simulink model "FlightCore_ROS2_loop"  (R2025b)
settings: Solver=FixedStepDiscrete  StartTime=0.0  StopTime=120  FixedStep=0.001  RelTol=1e-3
undefined symbols (not defined in the file): accel_bias_mps2, accel_body_mps2, angular_rate_body_radps, attitude_quat_wxyz, gyro_bias_radps, motor_cmd, position_ned_m, sequence, source_id, status, timestamp_sec, valid, velocity_ned_mps, wind_ned_mps
libraries: ros2lib x6
settings Model: DataDictionary=GlobalTypes.sldd  Creator=89447  LastModifiedBy=89447

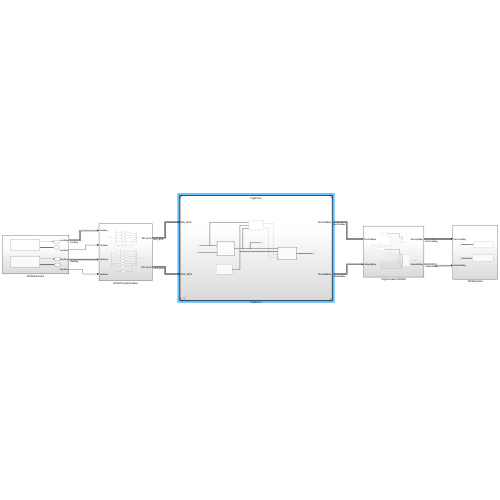
[thumbnail: Simulink's stored preview of the top-level diagram]
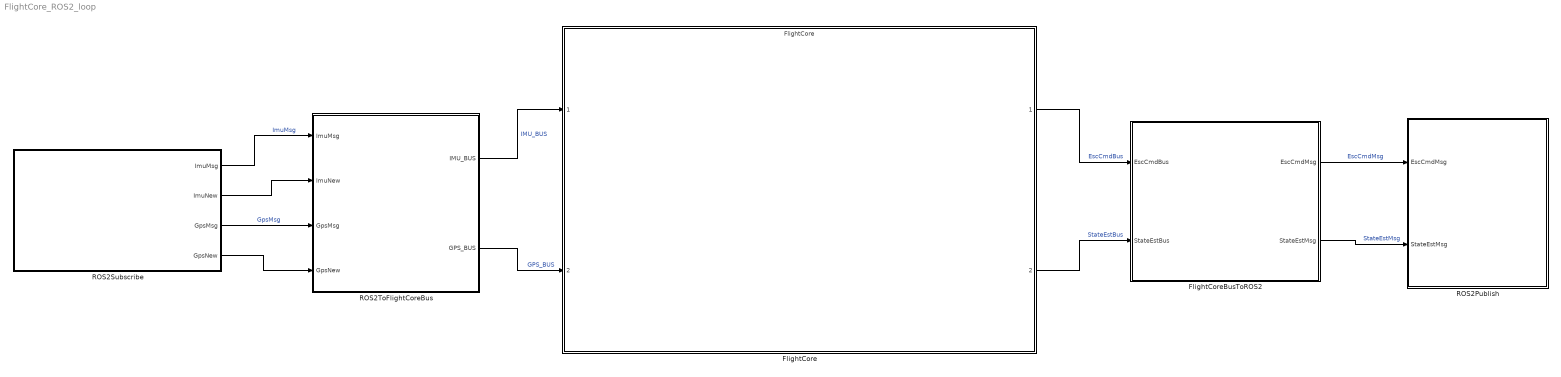
== system FlightCore_ROS2_loop ==
  FlightCore : ModelReference  ModelNameDialog=FlightCore  SimulationMode=Normal  ModelReferenceVersion=1.17
  FlightCoreBusToROS2 : Subsystem
  ROS2Publish : Subsystem
  ROS2Subscribe : Subsystem
  ROS2ToFlightCoreBus : Subsystem
  wires:
  ROS2Subscribe/3(GpsMsg) -> ROS2ToFlightCoreBus/3(GpsMsg)  "GpsMsg"
  ROS2Subscribe/1(ImuMsg) -> ROS2ToFlightCoreBus/1(ImuMsg)  "ImuMsg"
  ROS2ToFlightCoreBus/2(GPS_BUS) -> FlightCore/2  "GPS_BUS"
  ROS2ToFlightCoreBus/1(IMU_BUS) -> FlightCore/1  "IMU_BUS"
  FlightCore/2 -> FlightCoreBusToROS2/2(StateEstBus)  "StateEstBus"
  FlightCore/1 -> FlightCoreBusToROS2/1(EscCmdBus)  "EscCmdBus"
  FlightCoreBusToROS2/1(EscCmdMsg) -> ROS2Publish/1(EscCmdMsg)  "EscCmdMsg"
  FlightCoreBusToROS2/2(StateEstMsg) -> ROS2Publish/2(StateEstMsg)  "StateEstMsg"
  ROS2Subscribe/2(ImuNew) -> ROS2ToFlightCoreBus/2(ImuNew)
  ROS2Subscribe/4(GpsNew) -> ROS2ToFlightCoreBus/4(GpsNew)

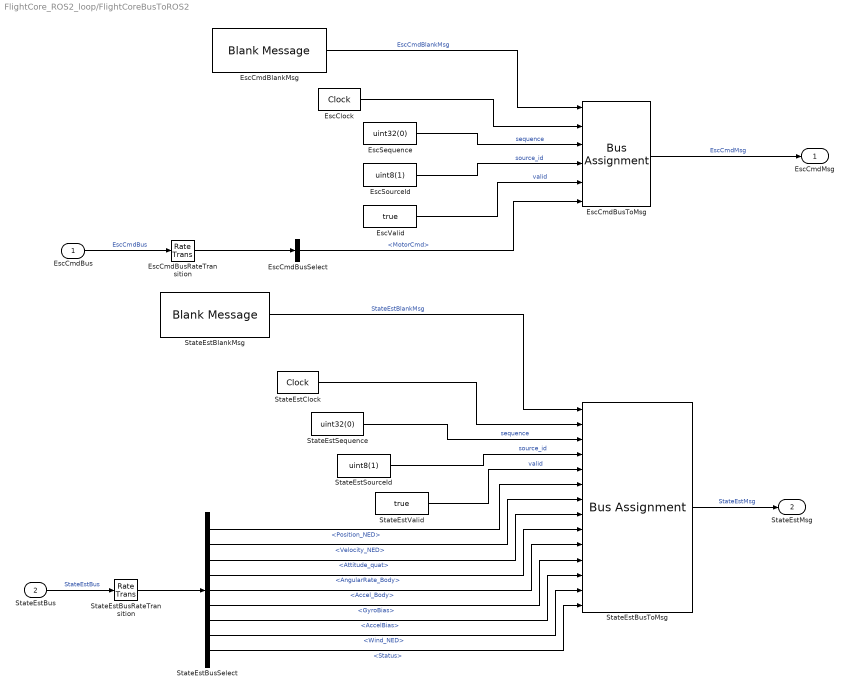
== system FlightCore_ROS2_loop/FlightCoreBusToROS2 ==
  EscCmdBus : Inport  OutDataTypeStr=Bus: EscCmdBus
  StateEstBus : Inport  Port=2  OutDataTypeStr=Bus: StateEstBus
  EscClock : DigitalClock  SampleTime=0.02
  EscCmdBlankMsg : ros2lib/Blank Message  messageClass=Message  entityType=flightcore_msgs/EscCmd  messageType=flightcore_msgs/EscCmd  SampleTime=0.02
  EscCmdBusRateTransition : RateTransition  OutPortSampleTime=0.02
  EscCmdBusSelect : BusSelector  OutputSignals=MotorCmd
  EscCmdBusToMsg : BusAssignment  AssignedSignals=timestamp_sec,sequence,source_id,valid,motor_cmd
  EscSequence : Constant  Value=uint32(0)  OutDataTypeStr=uint32
  EscSourceId : Constant  Value=uint8(1)  OutDataTypeStr=uint8
  EscValid : Constant  Value=true  OutDataTypeStr=boolean
  StateEstBlankMsg : ros2lib/Blank Message  messageClass=Message  entityType=flightcore_msgs/StateEst  messageType=flightcore_msgs/StateEst  SampleTime=0.02
  StateEstBusRateTransition : RateTransition  OutPortSampleTime=0.02
  StateEstBusSelect : BusSelector  OutputSignals=Position_NED,Velocity_NED,Attitude_quat,AngularRate_Body,Accel_Body,GyroBias,AccelBias,Wind_NED,Status
  StateEstBusToMsg : BusAssignment  AssignedSignals=timestamp_sec,sequence,source_id,valid,position_ned_m,velocity_ned_mps,attitude_quat_wxyz,angular_rate_body_radps,accel_body_mps2,gyro_bias_radps,accel_bias_mps2,wind_ned_mps,status
  StateEstClock : DigitalClock  SampleTime=0.02
  StateEstSequence : Constant  Value=uint32(0)  OutDataTypeStr=uint32
  StateEstSourceId : Constant  Value=uint8(1)  OutDataTypeStr=uint8
  StateEstValid : Constant  Value=true  OutDataTypeStr=boolean
  EscCmdMsg : Outport
  StateEstMsg : Outport  Port=2
  wires:
  EscCmdBlankMsg/1 -> EscCmdBusToMsg/1  "EscCmdBlankMsg"
  EscSequence/1 -> EscCmdBusToMsg/3  "sequence"
  EscSourceId/1 -> EscCmdBusToMsg/4  "source_id"
  EscValid/1 -> EscCmdBusToMsg/5  "valid"
  EscCmdBusSelect/1 -> EscCmdBusToMsg/6  "<MotorCmd>"
  EscCmdBusToMsg/1 -> EscCmdMsg/1  "EscCmdMsg"
  StateEstBlankMsg/1 -> StateEstBusToMsg/1  "StateEstBlankMsg"
  StateEstSequence/1 -> StateEstBusToMsg/3  "sequence"
  StateEstSourceId/1 -> StateEstBusToMsg/4  "source_id"
  StateEstValid/1 -> StateEstBusToMsg/5  "valid"
  StateEstBusSelect/1 -> StateEstBusToMsg/6  "<Position_NED>"
  StateEstBusSelect/2 -> StateEstBusToMsg/7  "<Velocity_NED>"
  StateEstBusSelect/3 -> StateEstBusToMsg/8  "<Attitude_quat>"
  StateEstBusSelect/4 -> StateEstBusToMsg/9  "<AngularRate_Body>"
  StateEstBusSelect/5 -> StateEstBusToMsg/10  "<Accel_Body>"
  StateEstBusSelect/6 -> StateEstBusToMsg/11  "<GyroBias>"
  StateEstBusSelect/7 -> StateEstBusToMsg/12  "<AccelBias>"
  StateEstBusSelect/8 -> StateEstBusToMsg/13  "<Wind_NED>"
  StateEstBusSelect/9 -> StateEstBusToMsg/14  "<Status>"
  StateEstBusToMsg/1 -> StateEstMsg/1  "StateEstMsg"
  EscCmdBus/1 -> EscCmdBusRateTransition/1  "EscCmdBus"
  EscCmdBusRateTransition/1 -> EscCmdBusSelect/1
  StateEstBus/1 -> StateEstBusRateTransition/1  "StateEstBus"
  StateEstBusRateTransition/1 -> StateEstBusSelect/1
  EscClock/1 -> EscCmdBusToMsg/2
  StateEstClock/1 -> StateEstBusToMsg/2

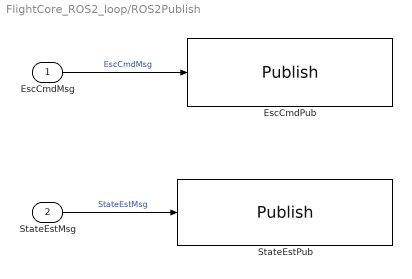
== system FlightCore_ROS2_loop/ROS2Publish ==
  EscCmdMsg : Inport
  StateEstMsg : Inport  Port=2
  EscCmdPub : ros2lib/Publish  topicSource=Specify your own  topic=/uav/actuator/esc_cmd  messageType=flightcore_msgs/EscCmd  QOSHistory=Keep last  QOSDepth=10  QOSReliability=Best effort  QOSDurability=Volatile  QOSDeadline=Inf  QOSLifespan=Inf  QOSLiveliness=Automatic  QOSLeaseDuration=Inf  QOSAvoidROSNamespaceConventions=off
  StateEstPub : ros2lib/Publish  topicSource=Specify your own  topic=/uav/estimator/state  messageType=flightcore_msgs/StateEst  QOSHistory=Keep last  QOSDepth=10  QOSReliability=Best effort  QOSDurability=Volatile  QOSDeadline=Inf  QOSLifespan=Inf  QOSLiveliness=Automatic  QOSLeaseDuration=Inf  QOSAvoidROSNamespaceConventions=off
  wires:
  EscCmdMsg/1 -> EscCmdPub/1  "EscCmdMsg"
  StateEstMsg/1 -> StateEstPub/1  "StateEstMsg"

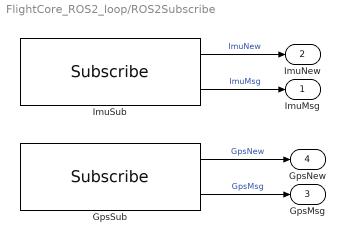
== system FlightCore_ROS2_loop/ROS2Subscribe ==
  GpsSub : ros2lib/Subscribe  topicSource=Specify your own  topic=/uav/sensors/gps  messageType=flightcore_msgs/Gps  sampleTime=0.1  QOSHistory=Keep last  QOSDepth=10  QOSReliability=Best effort  QOSDurability=Volatile  QOSDeadline=Inf  QOSLifespan=Inf  QOSLiveliness=Automatic  QOSLeaseDuration=Inf  QOSAvoidROSNamespaceConventions=off
  ImuSub : ros2lib/Subscribe  topicSource=Specify your own  topic=/uav/sensors/imu  messageType=flightcore_msgs/Imu  sampleTime=0.01  QOSHistory=Keep last  QOSDepth=10  QOSReliability=Best effort  QOSDurability=Volatile  QOSDeadline=Inf  QOSLifespan=Inf  QOSLiveliness=Automatic  QOSLeaseDuration=Inf  QOSAvoidROSNamespaceConventions=off
  ImuMsg : Outport
  ImuNew : Outport  Port=2
  GpsMsg : Outport  Port=3
  GpsNew : Outport  Port=4
  wires:
  ImuSub/2 -> ImuMsg/1  "ImuMsg"
  ImuSub/1 -> ImuNew/1  "ImuNew"
  GpsSub/2 -> GpsMsg/1  "GpsMsg"
  GpsSub/1 -> GpsNew/1  "GpsNew"

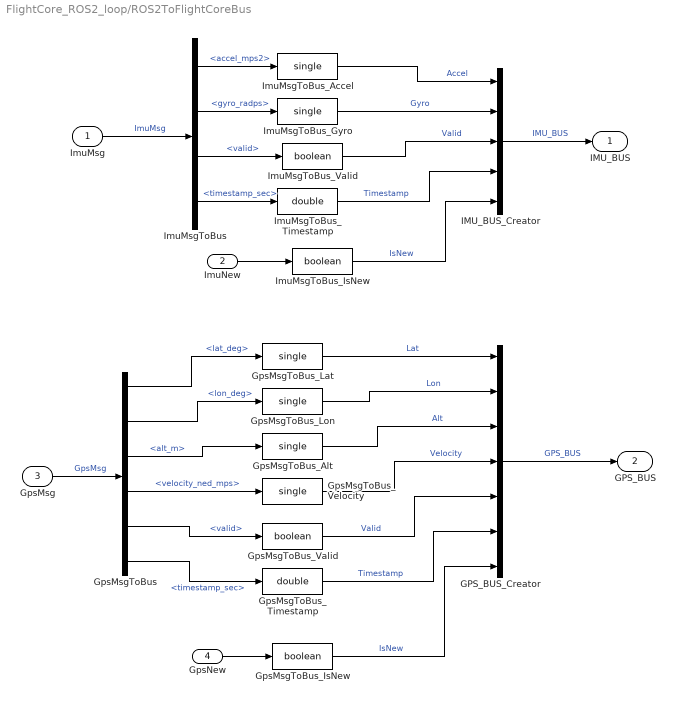
== system FlightCore_ROS2_loop/ROS2ToFlightCoreBus ==
  ImuMsg : Inport  OutDataTypeStr=Bus: SL_Bus_flightcore_msgs_Imu
  ImuNew : Inport  Port=2
  GpsMsg : Inport  Port=3  OutDataTypeStr=Bus: SL_Bus_flightcore_msgs_Gps
  GpsNew : Inport  Port=4
  GPS_BUS_Creator : BusCreator  Inputs=7  OutDataTypeStr=Bus: GPS_BUS
  GpsMsgToBus : BusSelector  OutputSignals=lat_deg,lon_deg,alt_m,velocity_ned_mps,valid,timestamp_sec
  GpsMsgToBus_Alt : DataTypeConversion  OutDataTypeStr=single  SaturateOnIntegerOverflow=off  RndMeth=Floor
  GpsMsgToBus_IsNew : DataTypeConversion  OutDataTypeStr=boolean  SaturateOnIntegerOverflow=off  RndMeth=Floor
  GpsMsgToBus_Lat : DataTypeConversion  OutDataTypeStr=single  SaturateOnIntegerOverflow=off  RndMeth=Floor
  GpsMsgToBus_Lon : DataTypeConversion  OutDataTypeStr=single  SaturateOnIntegerOverflow=off  RndMeth=Floor
  GpsMsgToBus_Timestamp : DataTypeConversion  OutDataTypeStr=double  SaturateOnIntegerOverflow=off  RndMeth=Floor
  GpsMsgToBus_Valid : DataTypeConversion  OutDataTypeStr=boolean  SaturateOnIntegerOverflow=off  RndMeth=Floor
  GpsMsgToBus_Velocity : DataTypeConversion  OutDataTypeStr=single  SaturateOnIntegerOverflow=off  RndMeth=Floor
  IMU_BUS_Creator : BusCreator  Inputs=5  OutDataTypeStr=Bus: IMU_BUS
  ImuMsgToBus : BusSelector  OutputSignals=accel_mps2,gyro_radps,valid,timestamp_sec
  ImuMsgToBus_Accel : DataTypeConversion  OutDataTypeStr=single  SaturateOnIntegerOverflow=off  RndMeth=Floor
  ImuMsgToBus_Gyro : DataTypeConversion  OutDataTypeStr=single  SaturateOnIntegerOverflow=off  RndMeth=Floor
  ImuMsgToBus_IsNew : DataTypeConversion  OutDataTypeStr=boolean  SaturateOnIntegerOverflow=off  RndMeth=Floor
  ImuMsgToBus_Timestamp : DataTypeConversion  OutDataTypeStr=double  SaturateOnIntegerOverflow=off  RndMeth=Floor
  ImuMsgToBus_Valid : DataTypeConversion  OutDataTypeStr=boolean  SaturateOnIntegerOverflow=off  RndMeth=Floor
  IMU_BUS : Outport  OutDataTypeStr=Bus: IMU_BUS
  GPS_BUS : Outport  Port=2  OutDataTypeStr=Bus: GPS_BUS
  wires:
  ImuMsg/1 -> ImuMsgToBus/1  "ImuMsg"
  ImuMsgToBus/1 -> ImuMsgToBus_Accel/1  "<accel_mps2>"
  ImuMsgToBus_Accel/1 -> IMU_BUS_Creator/1  "Accel"
  ImuMsgToBus/2 -> ImuMsgToBus_Gyro/1  "<gyro_radps>"
  ImuMsgToBus_Gyro/1 -> IMU_BUS_Creator/2  "Gyro"
  ImuMsgToBus/3 -> ImuMsgToBus_Valid/1  "<valid>"
  ImuMsgToBus_Valid/1 -> IMU_BUS_Creator/3  "Valid"
  ImuMsgToBus/4 -> ImuMsgToBus_Timestamp/1  "<timestamp_sec>"
  ImuMsgToBus_Timestamp/1 -> IMU_BUS_Creator/4  "Timestamp"
  IMU_BUS_Creator/1 -> IMU_BUS/1  "IMU_BUS"
  GpsMsg/1 -> GpsMsgToBus/1  "GpsMsg"
  GpsMsgToBus/1 -> GpsMsgToBus_Lat/1  "<lat_deg>"
  GpsMsgToBus_Lat/1 -> GPS_BUS_Creator/1  "Lat"
  GpsMsgToBus/2 -> GpsMsgToBus_Lon/1  "<lon_deg>"
  GpsMsgToBus_Lon/1 -> GPS_BUS_Creator/2  "Lon"
  GpsMsgToBus/3 -> GpsMsgToBus_Alt/1  "<alt_m>"
  GpsMsgToBus_Alt/1 -> GPS_BUS_Creator/3  "Alt"
  GpsMsgToBus/4 -> GpsMsgToBus_Velocity/1  "<velocity_ned_mps>"
  GpsMsgToBus_Velocity/1 -> GPS_BUS_Creator/4  "Velocity"
  GpsMsgToBus/5 -> GpsMsgToBus_Valid/1  "<valid>"
  GpsMsgToBus_Valid/1 -> GPS_BUS_Creator/5  "Valid"
  GpsMsgToBus/6 -> GpsMsgToBus_Timestamp/1  "<timestamp_sec>"
  GpsMsgToBus_Timestamp/1 -> GPS_BUS_Creator/6  "Timestamp"
  GPS_BUS_Creator/1 -> GPS_BUS/1  "GPS_BUS"
  ImuNew/1 -> ImuMsgToBus_IsNew/1
  ImuMsgToBus_IsNew/1 -> IMU_BUS_Creator/5  "IsNew"
  GpsNew/1 -> GpsMsgToBus_IsNew/1
  GpsMsgToBus_IsNew/1 -> GPS_BUS_Creator/7  "IsNew"
